simulink model "ZRM_U2A1"  (R2015a)
settings: Solver=ode45  StartTime=0.0  StopTime=10.0  RelTol=1e-3
values from neighbouring files (symbols this model uses):
  C = [5 4; 1 2]    [ZRM_U1.m]    (also in ZRM_U2.m = 3.3e-06; ZRM_Vorlesung1.m = [1 2 3;3 6 9;7 9 16])
  L = 50*10^(-6)    (= 5e-05)    [ZRM_U2.m]
  R = 10    [ZRM_U2.m]
libraries: simulink x1
settings Model: Creator=daniel  LastModifiedBy=daniel

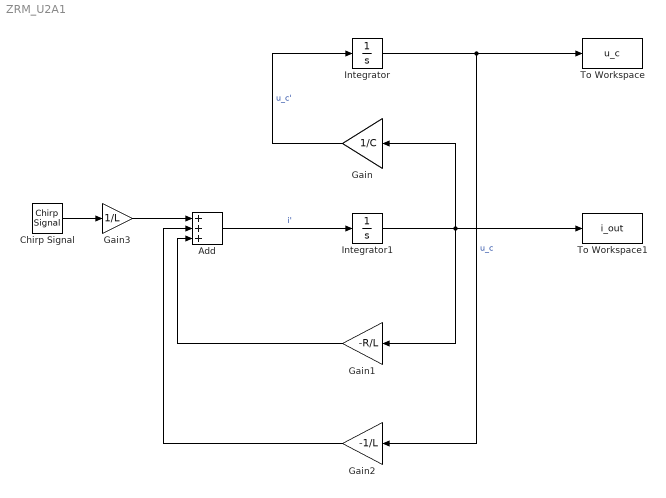
== system ZRM_U2A1 ==
  Add : Sum  Inputs=+++
  Chirp Signal : simulink/Sources/Chirp Signal  f1=init_freq  T=1000  f2=end_freq
  Gain : Gain  Gain=1/C
  Gain1 : Gain  Gain=-R/L
  Gain2 : Gain  Gain=-1/L
  Gain3 : Gain  Gain=1/L
  Integrator : Integrator
  Integrator1 : Integrator
  To Workspace : ToWorkspace  VariableName=u_c  SaveFormat=Structure With Time  SampleTime=-1
  To Workspace1 : ToWorkspace  VariableName=i_out  SaveFormat=Structure With Time  SampleTime=-1
  wires:
  Gain/1 -> Integrator/1  "u_c'"
  Add/1 -> Integrator1/1  "i'"
  Integrator1/1 -> Gain1/1, To Workspace1/1, Gain/1
  Gain1/1 -> Add/3
  Integrator/1 -> To Workspace/1, Gain2/1  "u_c"
  Gain2/1 -> Add/2
  Gain3/1 -> Add/1
  Chirp Signal/1 -> Gain3/1
